simulink model "Shravan_APS_SMC"  (R2019a)
settings: Solver=VariableStepAuto  StartTime=0.0  StopTime=20  RelTol=1e-3
libraries: Solver_SF x1
settings Model: Creator=srai25  LastModifiedBy=srai25
settings SolverCC: ZeroCrossAlgorithm=Adaptive
settings DebuggingCC: IgnoredZcDiagnostic=none

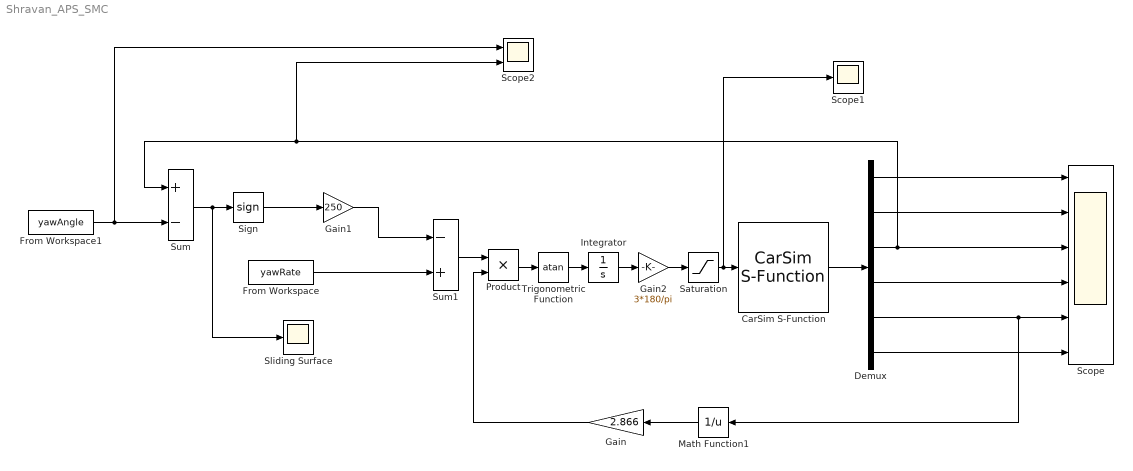
== system Shravan_APS_SMC ==
  CarSim S-Function : Solver_SF/CarSim S-Function  Priority=1  SIMFILE=simfile.sim
  Demux : Demux  Outputs=6
  From Workspace : FromWorkspace  VariableName=yawRate  SampleTime=0
  From Workspace1 : FromWorkspace  VariableName=yawAngle  SampleTime=0
  Gain : Gain  Gain=2.866
  Gain1 : Gain  Gain=250
  Gain2 : Gain  Gain=3*180/pi
  Integrator : Integrator  LimitOutput=on  UpperSaturationLimit=pi/2  LowerSaturationLimit=-pi/2
  Math Function1 : Math  Operator=reciprocal  SaturateOnIntegerOverflow=on
  Product : Product
  Saturation : Saturate  UpperLimit=280  LowerLimit=-280
  Scope : Scope  NumInputPorts=6
  Scope1 : Scope
  Scope2 : Scope  NumInputPorts=2
  Sign : Signum
  Sliding Surface : Scope
  Sum : Sum  Inputs=+-
  Sum1 : Sum  Inputs=-+
  Trigonometric Function : Trigonometry  Operator=atan  OutputSignalType=real
  wires:
  Trigonometric Function/1 -> Integrator/1
  CarSim S-Function/1 -> Demux/1
  Demux/5 -> Scope/5, Math Function1/1
  Math Function1/1 -> Gain/1
  Sum/1 -> Sliding Surface/1, Sign/1
  Sign/1 -> Gain1/1
  Gain1/1 -> Sum1/1
  From Workspace/1 -> Sum1/2
  Product/1 -> Trigonometric Function/1
  Sum1/1 -> Product/1
  Gain/1 -> Product/2
  Demux/1 -> Scope/1
  Demux/6 -> Scope/6
  Demux/4 -> Scope/4
  Demux/2 -> Scope/2
  From Workspace1/1 -> Sum/2, Scope2/1
  Demux/3 -> Scope/3, Scope2/2, Sum/1
  Integrator/1 -> Gain2/1
  Gain2/1 -> Saturation/1
  Saturation/1 -> Scope1/1, CarSim S-Function/1
